simulink model "arduino_lab_R2015a"  (R2015a)
settings: Solver=ode45  StartTime=0.0  StopTime=500  RelTol=1e-3
StartFcn:
  | clear all
libraries: realtime_pacer_lib x1
settings Model: Creator=johnh  LastModifiedBy=John Hedengren
settings DataIOCC: LimitDataPoints=off  SaveFormat=Dataset
settings HardwareCC: ProdBitPerPointer=64  ProdLargestAtomicFloat=Float  ProdIntDivRoundTo=Zero  ProdEndianess=LittleEndian  ProdHWDeviceType=Specified
settings ModelReferenceCC: PropagateSignalLabelsOutOfModel=on

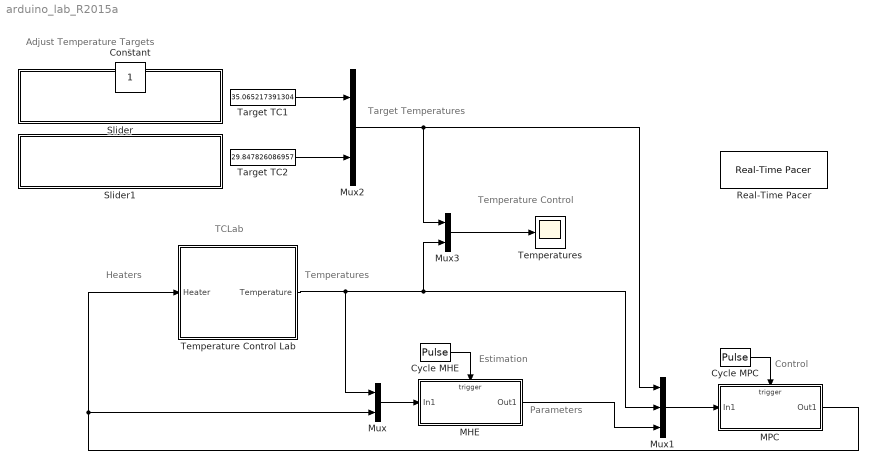
== system arduino_lab_R2015a ==
  note: Adjust Temperature Targets
  note: Temperature Control
  note: TCLab
  note: Heaters
  note: Estimation
  note: Control
  note: Temperatures
  note: Parameters
  note: Target Temperatures
  Cycle MHE : DiscretePulseGenerator  PulseType=Time based  Period=4  PulseWidth=5
  Cycle MPC : DiscretePulseGenerator  PulseType=Time based  Period=4  PulseWidth=5
  MHE : Subsystem  TreatAsAtomicUnit=on
  MPC : Subsystem  TreatAsAtomicUnit=on
  Mux : Mux  Inputs=2
  Mux1 : Mux  Inputs=3
  Mux2 : Mux  Inputs=2
  Mux3 : Mux  Inputs=2
  Real-Time Pacer : realtime_pacer_lib/Real-Time Pacer  simTimePerRealTime=1
  Slider : Subsystem  Description=Replaced Block  mask(Replaced Block){}
      mask help: This block has been replaced with an empty subsystem because it used functionality that is unavailable in Simulink R2015a.
      mask Display: fprintf('Replaced: %s\n','Dashboard Widget')
  Slider1 : Subsystem  Description=Replaced Block  mask(Replaced Block){}
      mask help: This block has been replaced with an empty subsystem because it used functionality that is unavailable in Simulink R2015a.
      mask Display: fprintf('Replaced: %s\n','Dashboard Widget')
  Target TC1 : Constant  Value=35.065217391304
  Target TC2 : Constant  Value=29.847826086957
  Temperature Control Lab : Subsystem
      mask Display: image('tclab.png');
  Temperatures : Scope
      settings: TimeRange=auto  LimitDataPoints=on  MaxDataPoints=5000  SaveToWorkspace=off  SaveName=ScopeData  YMin=13.11095  YMax=56.48827  SampleTime=-1  DataFormat=Array
  1 : Constant  IOType=siggen
  Constant : Constant  IOType=siggen
  wires:
  Cycle MPC/1 -> MPC/Trigger
  MPC/1(Out1) -> Mux/2, Temperature Control Lab/1(Heater)
  Temperature Control Lab/1(Temperature) -> Mux/1, Mux3/2, Mux1/2
  MHE/1(Out1) -> Mux1/3
  Mux/1 -> MHE/1(In1)
  Cycle MHE/1 -> MHE/Trigger
  Mux1/1 -> MPC/1(In1)
  Mux2/1 -> Mux1/1, Mux3/1
  Target TC1/1 -> Mux2/1
  Target TC2/1 -> Mux2/2
  Mux3/1 -> Temperatures/1

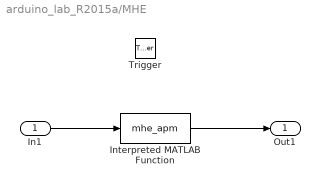
== system arduino_lab_R2015a/MHE ==
  In1 : Inport  LatchByDelayingOutsideSignal=on
  Trigger : TriggerPort
  Interpreted MATLAB Function : MATLABFcn  MATLABFcn=mhe_apm  OutputDimensions=5
  Out1 : Outport  InitialOutput=[2.5 5 0.005 0.0025 23]
  wires:
  In1/1 -> Interpreted MATLAB Function/1
  Interpreted MATLAB Function/1 -> Out1/1

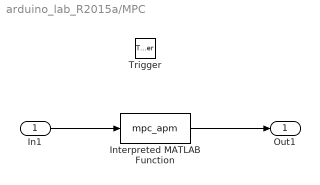
== system arduino_lab_R2015a/MPC ==
  In1 : Inport  LatchByDelayingOutsideSignal=on
  Trigger : TriggerPort
  Interpreted MATLAB Function : MATLABFcn  MATLABFcn=mpc_apm  OutputDimensions=2
  Out1 : Outport  InitialOutput=[0 0]
  wires:
  In1/1 -> Interpreted MATLAB Function/1
  Interpreted MATLAB Function/1 -> Out1/1

== system arduino_lab_R2015a/Slider ==

== system arduino_lab_R2015a/Slider1 ==

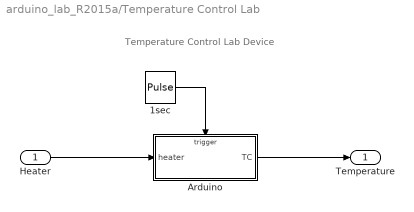
== system arduino_lab_R2015a/Temperature Control Lab ==
  note: Temperature Control Lab Device
  Heater : Inport
  1sec : DiscretePulseGenerator  PulseType=Time based  Period=1  PulseWidth=50
  Arduino : Subsystem  TreatAsAtomicUnit=on
  Temperature : Outport
  wires:
  1sec/1 -> Arduino/Trigger
  Arduino/1(TC) -> Temperature/1
  Heater/1 -> Arduino/1(heater)

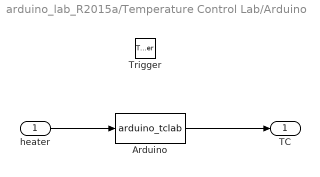
== system arduino_lab_R2015a/Temperature Control Lab/Arduino ==
  heater : Inport  LatchByDelayingOutsideSignal=on
  Trigger : TriggerPort
  Arduino : MATLABFcn  MATLABFcn=arduino_tclab
  TC : Outport  InitialOutput=[23 23]
  wires:
  heater/1 -> Arduino/1
  Arduino/1 -> TC/1
